simulink subsystem "LightSensor_Sim"  (R2020a)
settings: Solver=VariableStepAuto  StartTime=0.0  StopTime=10.0  RelTol=1e-3
values from neighbouring files (symbols this model uses):
  map = rgb2gray(map)    [test.m]
settings Model: Creator=Duncan  LastModifiedBy=abatra2

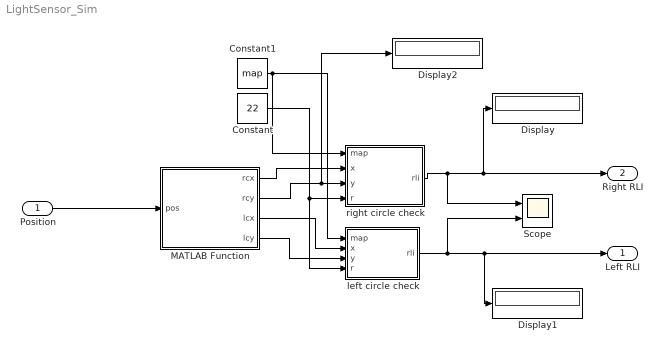
== system LightSensor_Sim ==
  Position : Inport
  Constant : Constant  Value=22
  Constant1 : Constant  Value=map
  Display : Display
  Display1 : Display
  Display2 : Display
  MATLAB Function : MATLAB Function  TreatAsAtomicUnit=on
  Scope : Scope  NumInputPorts=2
  left circle check : MATLAB Function  TreatAsAtomicUnit=on
  right circle check : MATLAB Function  TreatAsAtomicUnit=on
  Left RLI : Outport
  Right RLI : Outport  Port=2
  wires:
  Constant1/1 -> right circle check/1(map), left circle check/1(map)
  left circle check/1(rli) -> Scope/2, Left RLI/1, Display1/1
  right circle check/1(rli) -> Scope/1, Right RLI/1, Display/1
  MATLAB Function/1(rcx) -> right circle check/2(x)
  Position/1 -> MATLAB Function/1(pos)
  MATLAB Function/2(rcy) -> right circle check/3(y), Display2/1
  MATLAB Function/3(lcx) -> left circle check/2(x)
  MATLAB Function/4(lcy) -> left circle check/3(y)
  Constant/1 -> left circle check/4(r), right circle check/4(r)

== matlab function LightSensor_Sim/MATLAB Function ==
  data: pos input; rcx output; rcy output; lcx output; lcy output
function [rcx,rcy,lcx,lcy] = fcn(pos)
x = pos(1) + 0.06*cos(pos(3));
y = pos(2) + 0.06*sin(pos(3));
xScale = 1979.37;
yScale = -1925.58;
% xScale = 349.2718;
% yScale = -339.591;
topYReal = 2.936;
leftXReal = -1.9;
topYPixel = 943;
leftXPixel = 972;
% topYPixel = 168;
% leftXPixel = 166;
%pixel coords
x = round(leftXPixel + (xScale * (x-leftXReal)));
y = round(topYPixel + (yScale * (y-topYReal)));
lcy = floor(y-34*cos(pos(3)));
lcx = floor(x-34*sin(pos(3)));
rcy = floor(y+34*cos(pos(3)));
rcx = floor(x+34*sin(pos(3)));
% lcy = floor(y-6*cos(pos(3)));
% lcx = floor(x-6*sin(pos(3)));
% rcy = floor(y+6*cos(pos(3)));
% rcx = floor(x+6*sin(pos(3)));

end

== matlab function LightSensor_Sim/left circle check ==
  data: map input; rli output; x input; y input; r input
function rli = circle(map,x,y,r)
%x and y are the coordinates of the center of the circle
%r is the radius of the circle
region = map(y-r:y+r, x-r:x+r); %matlab indexes the opposite of images, select s square around the circle 
[MX,MY] = meshgrid(-r:r, -r:r);
mask = MX.^2 + MY.^2 <= r^2;
rli = sum(sum(region.*double(mask))) / sum(sum(mask));%sum(sum(mask));
rli = round(rli * .7 + 10);
end

== matlab function LightSensor_Sim/right circle check ==
  data: map input; rli output; x input; y input; r input
function rli = circle(map,x,y,r)
%x and y are the coordinates of the center of the circle
%r is the radius of the circle
region = map(y-r:y+r, x-r:x+r); %matlab indexes the opposite of images, select s square around the circle 
[MX,MY] = meshgrid(-r:r, -r:r);
mask = MX.^2 + MY.^2 <= r^2;
rli = sum(sum(region.*double(mask))) / sum(sum(mask));%sum(sum(mask));
rli = round(rli*.7 + 10);
end
